simulink library "UAVdesign_net"  (Simulink 7.7)
settings: Solver=ode45  SolverMode=SingleTasking  StartTime=0.0  StopTime=10.0  RelTol=1e-3
undefined symbols (not defined in the file or in its folder): alpha_IERA_IELA_IELA, R_IERA_RA_RA
libraries: UAVdesign_net x75, simulink x13
(part 7 of 8)

== system UAVdesign_net/Vehicle Models/Helicopter Model/RA to IELA CG computation/RA to IELA 4 ==
  Geometry : Inport  OutDataTypeStr=Bus: GeometryParameters
  CG_RA_RA : Inport  Port=2
  Bus Selector : BusSelector  OutputSignals=R_IERA_RA_RA,alpha_IERA_IELA_IELA,m,I_IERA
  Dot Product : simulink/Math Operations/Dot Product  InputSameDT=on  OutDataType=sfix(16)  OutScaling=2^-10  DoSatur=off
  Identity matrix : Constant  Value=[1 0 0; 0 1 0; 0 0 1]
  Product : Product  RndMeth=Zero
  Product1 : Product  RndMeth=Zero
  Product2 : Product  Multiplication=Matrix(*)  RndMeth=Zero
  Product3 : Product  RndMeth=Zero
  RA to IELA1 : Subsystem
  Reshape : Reshape  OutputDimensionality=Column vector (2-D)
  Reshape1 : Reshape  OutputDimensionality=Row vector (2-D)
  Rotate to IELA : Product  Inputs=3  Multiplication=Matrix(*)  RndMeth=Zero
  Rotation Matrix from IELA to IERA : UAVdesign_net/Utilities/Axes/Euler Rotation Matrix from Earth to Body  SystemSampleTime=-1
  Sum : Sum  Inputs=-+|
  Sum1 : Sum  Inputs=+|+
  Sum2 : Sum  Inputs=|+-
  Transpose : Subsystem
      mask Display: disp('A^T', 'texmode', 'on')
  R_IELA_B_B : Outport
  alpha_IERA_IELA : Outport  Port=2
  T_IERA_IELA : Outport  Port=3
  T_IELA_IERA : Outport  Port=4
  mass_distance : Outport  Port=5
  m : Outport  Port=6
  In_CG : Outport  Port=7
  wires:
  Bus Selector/4 -> Rotate to IELA/2  "<I_IERA>"
  Rotate to IELA/1 -> Sum1/1
  Transpose/1(Out) -> Rotate to IELA/3, T_IELA_IERA/1
  Rotation Matrix from IELA to IERA/1 -> Rotate to IELA/1, T_IERA_IELA/1, Transpose/1(In)
  RA to IELA1/1(IELA) -> R_IELA_B_B/1, Reshape/1, Reshape1/1, Dot Product/2, Dot Product/1
  CG_RA_RA/1 -> Sum/1
  Sum1/1 -> In_CG/1
  Product/1 -> mass_distance/1
  Geometry/1 -> Bus Selector/1
  Sum2/1 -> Product1/2
  Product2/1 -> Sum2/2
  Product3/1 -> Sum2/1
  Identity matrix/1 -> Product3/1
  Dot Product/1 -> Product3/2
  Reshape1/1 -> Product2/2
  Reshape/1 -> Product2/1
  Product1/1 -> Sum1/2
  Sum/1 -> RA to IELA1/1(RA)
  Bus Selector/3 -> m/1, Product1/1, Product/2  "<m>"
  Bus Selector/2 -> Rotation Matrix from IELA to IERA/1, alpha_IERA_IELA/1  "<alpha_IERA_IELA_IELA>"
  Bus Selector/1 -> Sum/2, Product/1  "<R_IERA_RA_RA>"

== system UAVdesign_net/Vehicle Models/Helicopter Model/RA to IELA CG computation/RA to IELA 5 ==
  Geometry : Inport  OutDataTypeStr=Bus: GeometryParameters
  CG_RA_RA : Inport  Port=2
  Bus Selector : BusSelector  OutputSignals=R_IERA_RA_RA,alpha_IERA_IELA_IELA,m,I_IERA
  Dot Product : simulink/Math Operations/Dot Product  InputSameDT=on  OutDataType=sfix(16)  OutScaling=2^-10  DoSatur=off
  Identity matrix : Constant  Value=[1 0 0; 0 1 0; 0 0 1]
  Product : Product  RndMeth=Zero
  Product1 : Product  RndMeth=Zero
  Product2 : Product  Multiplication=Matrix(*)  RndMeth=Zero
  Product3 : Product  RndMeth=Zero
  RA to IELA1 : Subsystem
  Reshape : Reshape  OutputDimensionality=Column vector (2-D)
  Reshape1 : Reshape  OutputDimensionality=Row vector (2-D)
  Rotate to IELA : Product  Inputs=3  Multiplication=Matrix(*)  RndMeth=Zero
  Rotation Matrix from IELA to IERA : UAVdesign_net/Utilities/Axes/Euler Rotation Matrix from Earth to Body  SystemSampleTime=-1
  Sum : Sum  Inputs=-+|
  Sum1 : Sum  Inputs=+|+
  Sum2 : Sum  Inputs=|+-
  Transpose : Subsystem
      mask Display: disp('A^T', 'texmode', 'on')
  R_IELA_B_B : Outport
  alpha_IERA_IELA : Outport  Port=2
  T_IERA_IELA : Outport  Port=3
  T_IELA_IERA : Outport  Port=4
  mass_distance : Outport  Port=5
  m : Outport  Port=6
  In_CG : Outport  Port=7
  wires:
  Bus Selector/1 -> Product/1, Sum/2  "<R_IERA_RA_RA>"
  Bus Selector/2 -> alpha_IERA_IELA/1, Rotation Matrix from IELA to IERA/1  "<alpha_IERA_IELA_IELA>"
  Bus Selector/3 -> Product/2, Product1/1, m/1  "<m>"
  Sum/1 -> RA to IELA1/1(RA)
  Product1/1 -> Sum1/2
  Reshape/1 -> Product2/1
  Reshape1/1 -> Product2/2
  Dot Product/1 -> Product3/2
  Identity matrix/1 -> Product3/1
  Product3/1 -> Sum2/1
  Product2/1 -> Sum2/2
  Sum2/1 -> Product1/2
  Geometry/1 -> Bus Selector/1
  Product/1 -> mass_distance/1
  Sum1/1 -> In_CG/1
  CG_RA_RA/1 -> Sum/1
  RA to IELA1/1(IELA) -> Dot Product/1, Dot Product/2, Reshape1/1, Reshape/1, R_IELA_B_B/1
  Rotation Matrix from IELA to IERA/1 -> Transpose/1(In), T_IERA_IELA/1, Rotate to IELA/1
  Transpose/1(Out) -> T_IELA_IERA/1, Rotate to IELA/3
  Rotate to IELA/1 -> Sum1/1
  Bus Selector/4 -> Rotate to IELA/2  "<I_IERA>"

== system UAVdesign_net/Vehicle Models/Helicopter Model/RA to IELA CG computation/RA to IELA 6 ==
  Geometry : Inport  OutDataTypeStr=Bus: GeometryParameters
  CG_RA_RA : Inport  Port=2
  Bus Selector : BusSelector  OutputSignals=R_IERA_RA_RA,alpha_IERA_IELA_IELA,m,I_IERA
  Dot Product : simulink/Math Operations/Dot Product  InputSameDT=on  OutDataType=sfix(16)  OutScaling=2^-10  DoSatur=off
  Identity matrix : Constant  Value=[1 0 0; 0 1 0; 0 0 1]
  Product : Product  RndMeth=Zero
  Product1 : Product  RndMeth=Zero
  Product2 : Product  Multiplication=Matrix(*)  RndMeth=Zero
  Product3 : Product  RndMeth=Zero
  RA to IELA1 : Subsystem
  Reshape : Reshape  OutputDimensionality=Column vector (2-D)
  Reshape1 : Reshape  OutputDimensionality=Row vector (2-D)
  Rotate to IELA : Product  Inputs=3  Multiplication=Matrix(*)  RndMeth=Zero
  Rotation Matrix from IELA to IERA : UAVdesign_net/Utilities/Axes/Euler Rotation Matrix from Earth to Body  SystemSampleTime=-1
  Sum : Sum  Inputs=-+|
  Sum1 : Sum  Inputs=+|+
  Sum2 : Sum  Inputs=|+-
  Transpose : Subsystem
      mask Display: disp('A^T', 'texmode', 'on')
  R_IELA_B_B : Outport
  alpha_IERA_IELA : Outport  Port=2
  T_IERA_IELA : Outport  Port=3
  T_IELA_IERA : Outport  Port=4
  mass_distance : Outport  Port=5
  m : Outport  Port=6
  In_CG : Outport  Port=7
  wires:
  Bus Selector/4 -> Rotate to IELA/2  "<I_IERA>"
  Rotate to IELA/1 -> Sum1/1
  Transpose/1(Out) -> Rotate to IELA/3, T_IELA_IERA/1
  Rotation Matrix from IELA to IERA/1 -> Rotate to IELA/1, T_IERA_IELA/1, Transpose/1(In)
  RA to IELA1/1(IELA) -> R_IELA_B_B/1, Reshape/1, Reshape1/1, Dot Product/2, Dot Product/1
  CG_RA_RA/1 -> Sum/1
  Sum1/1 -> In_CG/1
  Product/1 -> mass_distance/1
  Geometry/1 -> Bus Selector/1
  Sum2/1 -> Product1/2
  Product2/1 -> Sum2/2
  Product3/1 -> Sum2/1
  Identity matrix/1 -> Product3/1
  Dot Product/1 -> Product3/2
  Reshape1/1 -> Product2/2
  Reshape/1 -> Product2/1
  Product1/1 -> Sum1/2
  Sum/1 -> RA to IELA1/1(RA)
  Bus Selector/3 -> m/1, Product1/1, Product/2  "<m>"
  Bus Selector/2 -> Rotation Matrix from IELA to IERA/1, alpha_IERA_IELA/1  "<alpha_IERA_IELA_IELA>"
  Bus Selector/1 -> Sum/2, Product/1  "<R_IERA_RA_RA>"

== system UAVdesign_net/Vehicle Models/Quad-Rotor Model (Momentum)/Fuselage/CG to IELA ==
  R_IELA-B|B : Inport
  V_B-E|B : Inport  Port=2
  omega_B_E|B : Inport  Port=3
  3x3 Cross Product : UAVdesign_net/Utilities/Math/3x3 Cross Product  SystemSampleTime=-1
  Sum : Sum  Inputs=++|
  V_IELA-E|IELA : Outport
  omega_IELA-E|IELA : Outport  Port=2
  wires:
  Sum/1 -> V_IELA-E|IELA/1
  V_B-E|B/1 -> Sum/1
  3x3 Cross Product/1 -> Sum/2
  R_IELA-B|B/1 -> 3x3 Cross Product/2
  omega_B_E|B/1 -> omega_IELA-E|IELA/1, 3x3 Cross Product/1

== system UAVdesign_net/Vehicle Models/Quad-Rotor Model (Momentum)/Fuselage/Fuselage Model (IERA) ==
  Parameters : Inport
  Environment : Inport  Port=2
  V_A : Inport  Port=3
  omega_A : Inport  Port=4
  V_W : Inport  Port=5
  omega_W : Inport  Port=6
  Fuselage Forces and Moments : Subsystem
      mask Display:
      | port_label('input', 1, 'Parameters', 'texmode', 'on')
      | port_label('input', 2, 'Environment', 'texmode', 'on')
      | port_label('input', 3, 'V_{A|WRA}', 'texmode', 'on')
      | port_label('input', 4, '\omega_{A|WRA}', 'texmode', 'on')
      | 
      | port_label('output', 1, 'FM_{A}', 'texmode', 'on')
  Fuselage Self-Influence : Subsystem
      mask Display:
      | port_label('input', 1, 'Parameters', 'texmode', 'on')
      | port_label('input', 2, 'Environment', 'texmode', 'on')
      | port_label('input', 3, 'V_{A|IERA}', 'texmode', 'on')
      | port_label('input', 4, '\omega_{A|IERA}', 'texmode', 'on')
      | port_label('input', 5, 'FM_{A|IERA}', 'texmode', 'on')
      | 
      | port_label('output', 1, 'd_{k|IERA}', 'texmode', 'on')
  Terminator : Terminator
  Terminator1 : Terminator
  Zero inertial : Constant  Value=[0 0 0 0 0 0]
  FM_I : Outport
  FM_A : Outport  Port=2
  d (k) : Outport  Port=3
  wires:
  Fuselage Self-Influence/1(d (k)) -> d (k)/1
  Fuselage Forces and Moments/1(FM_A) -> Fuselage Self-Influence/5(FM_A), FM_A/1
  Zero inertial/1 -> FM_I/1
  omega_W/1 -> Terminator1/1
  V_W/1 -> Terminator/1
  omega_A/1 -> Fuselage Forces and Moments/4(omega_A), Fuselage Self-Influence/4(omega_A)
  V_A/1 -> Fuselage Forces and Moments/3(V_A), Fuselage Self-Influence/3(V_A)
  Environment/1 -> Fuselage Forces and Moments/2(Environment), Fuselage Self-Influence/2(Environment)
  Parameters/1 -> Fuselage Forces and Moments/1(Parameters), Fuselage Self-Influence/1(Parameters)

== system UAVdesign_net/Vehicle Models/Quad-Rotor Model (Momentum)/Fuselage/IELA to CG ==
  R_IELA_B_B : Inport
  FM_IELA : Inport  Port=2
  3x3 Cross Product : UAVdesign_net/Utilities/Math/3x3 Cross Product  SystemSampleTime=-1
  Demux : Demux  Outputs=2
  Mux : Mux  Inputs=2
  Sum : Sum  Inputs=++|
  FM_B : Outport
  wires:
  3x3 Cross Product/1 -> Sum/1
  Sum/1 -> Mux/2
  Demux/2 -> Sum/2
  R_IELA_B_B/1 -> 3x3 Cross Product/1
  Demux/1 -> 3x3 Cross Product/2, Mux/1
  Mux/1 -> FM_B/1
  FM_IELA/1 -> Demux/1

== system UAVdesign_net/Vehicle Models/Quad-Rotor Model (Momentum)/Fuselage/IELA to IERA ==
  T_IERA_IELA : Inport
  V_A_IELA : Inport  Port=2
  omega_A_IELA : Inport  Port=3
  V_W_IELA : Inport  Port=4
  omega_W_IELA : Inport  Port=5
  1D : Reshape
  Demux : Demux
  Product : Product  Multiplication=Matrix(*)  RndMeth=Zero
  Vector Concatenate : Concatenate  NumInputs=4  Mode=Multidimensional array  ConcatenateDimension=2
  V_A_IERA : Outport
  omega_A_IERA : Outport  Port=2
  V_W_IERA : Outport  Port=3
  omega_W_IERA : Outport  Port=4
  wires:
  omega_W_IELA/1 -> Vector Concatenate/4
  V_W_IELA/1 -> Vector Concatenate/3
  Demux/4 -> omega_W_IERA/1
  Demux/3 -> V_W_IERA/1
  Demux/2 -> omega_A_IERA/1
  Demux/1 -> V_A_IERA/1
  1D/1 -> Demux/1
  Product/1 -> 1D/1
  Vector Concatenate/1 -> Product/2
  omega_A_IELA/1 -> Vector Concatenate/2
  V_A_IELA/1 -> Vector Concatenate/1
  T_IERA_IELA/1 -> Product/1

== system UAVdesign_net/Vehicle Models/Quad-Rotor Model (Momentum)/Fuselage/IERA to IELA ==
  T_IELA_IERA : Inport
  FM_I_IERA : Inport  Port=2
  FM_A_IERA : Inport  Port=3
  d_IERA : Inport  Port=4
  1D : Reshape
  Demux : Demux  Outputs=[6 6 3]
  Demux1 : Demux  Outputs=2
  Demux2 : Demux  Outputs=2
  Product : Product  Multiplication=Matrix(*)  RndMeth=Zero
  Signal Specification{,1..4} (5 alike) : SignalSpecification  Dimensions=3
  Vector Concatenate : Concatenate  NumInputs=5  Mode=Multidimensional array  ConcatenateDimension=2
  FM_I_IELA : Outport
  FM_A_IELA : Outport  Port=2
  d_IELA : Outport  Port=3
  wires:
  Signal Specification4/1 -> Vector Concatenate/5
  Signal Specification3/1 -> Vector Concatenate/4
  Signal Specification2/1 -> Vector Concatenate/3
  Signal Specification1/1 -> Vector Concatenate/2
  Signal Specification/1 -> Vector Concatenate/1
  FM_A_IERA/1 -> Demux2/1
  Demux2/2 -> Signal Specification3/1
  Demux2/1 -> Signal Specification2/1
  Demux1/1 -> Signal Specification/1
  Demux1/2 -> Signal Specification1/1
  FM_I_IERA/1 -> Demux1/1
  d_IERA/1 -> Signal Specification4/1
  Demux/3 -> d_IELA/1
  Demux/2 -> FM_A_IELA/1
  Demux/1 -> FM_I_IELA/1
  1D/1 -> Demux/1
  Product/1 -> 1D/1
  Vector Concatenate/1 -> Product/2
  T_IELA_IERA/1 -> Product/1

== system UAVdesign_net/Vehicle Models/Quad-Rotor Model (Momentum)/Fuselage/Transpose ==
  In : Inport
  Permute Dimensions : PermuteDimensions
  Out : Outport
  wires:
  In/1 -> Permute Dimensions/1
  Permute Dimensions/1 -> Out/1

== system UAVdesign_net/Vehicle Models/Quad-Rotor Model (Momentum)/RA to IELA CG computation/Body Coordinates Computation ==
  Geometry : Inport
  R_CG_RA_RA : Inport  Port=2
  Assignment : Assignment  NumberOfDimensions=2  IndexMode=Zero-based  OutputInitialize=Specify size for each dimension in table  IndexOptions=Assign all,Starting index (port)  Indices=1,1  OutputSizes=3,3*6
  Assignment1 : Assignment  IndexMode=Zero-based  OutputInitialize=Specify size for each dimension in table  IndexOptions=Starting index (port)  Indices=1  OutputSizes=3*6
  Bus Selector : BusSelector  OutputSignals=COMMON.R_IERA_RA_RA,COMMON.alpha_IERA_IELA_IELA,COMMON.m,COMMON.I_IERA
  For Iterator : ForIterator  ResetStates=reset  IterationLimit=6  IndexMode=Zero-based
  Gain{,1..4} (5 alike) : Gain  Gain=3  OutDataTypeStr=uint32
  RA to IELA : Subsystem
  Rotation Matrix from IELA to IERA : UAVdesign_net/Utilities/Axes/Euler Rotation Matrix from Earth to Body  SystemSampleTime=-1
  Selector : Selector  IndexMode=Zero-based  InputPortWidth=3*6  IndexOptions=Starting index (port)  Indices=[1 3]  OutputSizes=3
  Selector1 : Selector  IndexMode=Zero-based  InputPortWidth=3*6  IndexOptions=Starting index (port)  Indices=[1 3]  OutputSizes=3
  Selector2 : Selector  IndexMode=Zero-based  InputPortWidth=6  IndexOptions=Starting index (port)  Indices=[1 3]  OutputSizes=1
  Selector3 : Selector  NumberOfDimensions=2  IndexMode=Zero-based  InputPortWidth=6  IndexOptions=Select all,Starting index (port)  Indices=[1 3],1  OutputSizes=1,3
  Sum : Sum  Inputs=|++
  Unit Delay : UnitDelay  SampleTime=-1
  R_IERA_B_B : Outport
  T_IERA_IELA : Outport  Port=2
  Inb : Outport  Port=3
  wires:
  Sum/1 -> Unit Delay/1, Inb/1
  Unit Delay/1 -> Sum/1
  RA to IELA/2(In_CG) -> Sum/2
  Gain/1 -> Selector/2
  Gain1/1 -> Selector1/2
  For Iterator/1 -> Gain/1, Gain1/1, Selector2/2, Gain2/1, Gain3/1, Gain4/1
  Bus Selector/3 -> Selector2/1  "<m>"
  Geometry/1 -> Bus Selector/1
  Bus Selector/1 -> Selector/1  "<R_IERA_RA_RA>"
  Bus Selector/2 -> Selector1/1  "<alpha_IERA_IELA_IELA>"
  Rotation Matrix from IELA to IERA/1 -> RA to IELA/5(T_IERA_IELA), Assignment/1
  Bus Selector/4 -> Selector3/1  "<I_IERA>"
  Gain2/1 -> Selector3/2
  Selector1/1 -> Rotation Matrix from IELA to IERA/1
  Selector3/1 -> RA to IELA/4(I_IERA)
  Selector2/1 -> RA to IELA/3(m)
  Selector/1 -> RA to IELA/2(R_IERA_RA_RA)
  R_CG_RA_RA/1 -> RA to IELA/1(R_CG_RA_RA)
  Assignment/1 -> T_IERA_IELA/1
  Gain3/1 -> Assignment/2
  Gain4/1 -> Assignment1/2
  Assignment1/1 -> R_IERA_B_B/1
  RA to IELA/1(R_IELA_B_B) -> Assignment1/1

== system UAVdesign_net/Vehicle Models/Quad-Rotor Model (Momentum)/RA to IELA CG computation/GC Computation ==
  Geometry : Inport
  Bus Selector : BusSelector  OutputSignals=COMMON.R_IERA_RA_RA,COMMON.m
  For Iterator : ForIterator  ResetStates=reset  IterationLimit=6  IndexMode=Zero-based
  Gain : Gain  Gain=3  OutDataTypeStr=uint32
  Product : Product  RndMeth=Zero
  Selector : Selector  IndexMode=Zero-based  InputPortWidth=3*6  IndexOptions=Starting index (port)  Indices=[1 3]  OutputSizes=3
  Selector2 : Selector  IndexMode=Zero-based  InputPortWidth=6  IndexOptions=Starting index (port)  Indices=[1 3]  OutputSizes=1
  Sum : Sum  Inputs=|++
  Sum2 : Sum  Inputs=|++
  Unit Delay : UnitDelay  SampleTime=-1
  Unit Delay2 : UnitDelay  X0=[0 0 0]  SampleTime=-1
  R_CG_RA_RA_m : Outport
  mass : Outport  Port=2
  wires:
  Unit Delay/1 -> Sum/1
  Sum/1 -> mass/1, Unit Delay/1
  Unit Delay2/1 -> Sum2/1
  Sum2/1 -> Unit Delay2/1, R_CG_RA_RA_m/1
  Product/1 -> Sum2/2
  Selector2/1 -> Sum/2, Product/2
  Selector/1 -> Product/1
  Gain/1 -> Selector/2
  For Iterator/1 -> Gain/1, Selector2/2
  Bus Selector/2 -> Selector2/1  "<m>"
  Geometry/1 -> Bus Selector/1
  Bus Selector/1 -> Selector/1  "<R_IERA_RA_RA>"

== system UAVdesign_net/Subsystem Models/Fin/Fin Model (IERA)/Fin/Fin Forces and Moments ==
  Parameters : Inport  OutDataTypeStr=Bus: FinParameters
  Environment : Inport  Port=2  OutDataTypeStr=Bus: Environment
  V_A : Inport  Port=3
  omega_A : Inport  Port=4
  Fin Forces and Moments (WRA axes) : Stateflow chart  TreatAsAtomicUnit=on
  FM_A : Outport
  wires:
  Parameters/1 -> Fin Forces and Moments (WRA axes)/1(Parameters)
  Environment/1 -> Fin Forces and Moments (WRA axes)/2(Environment)
  V_A/1 -> Fin Forces and Moments (WRA axes)/3(va)
  omega_A/1 -> Fin Forces and Moments (WRA axes)/4(oma)
  Fin Forces and Moments (WRA axes)/1(FM_A) -> FM_A/1

== system UAVdesign_net/Subsystem Models/Fin/Fin Model (IERA)/Fin/IERA to MAC ==
  R_xW-IERA|IERA : Inport
  V_A|IERA : Inport  Port=2
  omega_A|IERA : Inport  Port=3
  3x3 Cross Product : UAVdesign_net/Utilities/Math/3x3 Cross Product  SystemSampleTime=-1
  Sum : Sum  Inputs=++|
  V_A|MAC : Outport
  omega_A|MAC : Outport  Port=2
  wires:
  Sum/1 -> V_A|MAC/1
  V_A|IERA/1 -> Sum/1
  3x3 Cross Product/1 -> Sum/2
  R_xW-IERA|IERA/1 -> 3x3 Cross Product/2
  omega_A|IERA/1 -> omega_A|MAC/1, 3x3 Cross Product/1

== system UAVdesign_net/Subsystem Models/Fin/Fin Model (IERA)/Fin/MAC to IERA ==
  R_MAC_IERA_IERA : Inport
  FM_MAC : Inport  Port=2
  3x3 Cross Product : UAVdesign_net/Utilities/Math/3x3 Cross Product  SystemSampleTime=-1
  Demux : Demux  Outputs=2
  Mux : Mux  Inputs=2
  Sum : Sum  Inputs=++|
  FM_IERA : Outport
  wires:
  FM_MAC/1 -> Demux/1
  Mux/1 -> FM_IERA/1
  Demux/1 -> Mux/1, 3x3 Cross Product/2
  R_MAC_IERA_IERA/1 -> 3x3 Cross Product/1
  Demux/2 -> Sum/2
  Sum/1 -> Mux/2
  3x3 Cross Product/1 -> Sum/1

== system UAVdesign_net/Subsystem Models/Fin/Fin Model (IERA)/Fin/MAC to WRA (Half Wing) ==
  T_WRA_MAC : Inport
  V_A_MAC : Inport  Port=2
  omega_A_MAC : Inport  Port=3
  1D : Reshape
  Demux : Demux  Outputs=2
  Product : Product  Multiplication=Matrix(*)  RndMeth=Zero
  Vector Concatenate : Concatenate  Mode=Multidimensional array  ConcatenateDimension=2
  V_A_WRA : Outport
  omega_A_WRA : Outport  Port=2
  wires:
  Demux/2 -> omega_A_WRA/1
  Demux/1 -> V_A_WRA/1
  1D/1 -> Demux/1
  Product/1 -> 1D/1
  Vector Concatenate/1 -> Product/2
  omega_A_MAC/1 -> Vector Concatenate/2
  V_A_MAC/1 -> Vector Concatenate/1
  T_WRA_MAC/1 -> Product/1

== system UAVdesign_net/Subsystem Models/Fin/Fin Model (IERA)/Fin/WRA to MAC ==
  T_IERA_WM : Inport
  FM_A_WM : Inport  Port=2
  1D : Reshape
  Demux1 : Demux  Outputs=2
  Product : Product  Multiplication=Matrix(*)  RndMeth=Zero
  Vector Concatenate : Concatenate  Mode=Multidimensional array  ConcatenateDimension=2
  FM_A_IERA : Outport
  wires:
  T_IERA_WM/1 -> Product/1
  Vector Concatenate/1 -> Product/2
  Product/1 -> 1D/1
  1D/1 -> FM_A_IERA/1
  Demux1/1 -> Vector Concatenate/1
  Demux1/2 -> Vector Concatenate/2
  FM_A_WM/1 -> Demux1/1

== system UAVdesign_net/Subsystem Models/Wing/Wing Model (IERA)/Left Wing/Half Wing Forces and Moments ==
  Parameters : Inport  OutDataTypeStr=Bus: FinParameters
  Environment : Inport  Port=2  OutDataTypeStr=Bus: Environment
  V_A : Inport  Port=3
  omega_A : Inport  Port=4
  Wing Forces and Moments (WRA axes) : Stateflow chart  TreatAsAtomicUnit=on
  FM_A : Outport
  wires:
  Parameters/1 -> Wing Forces and Moments (WRA axes)/1(Parameters)
  Environment/1 -> Wing Forces and Moments (WRA axes)/2(Environment)
  V_A/1 -> Wing Forces and Moments (WRA axes)/3(va)
  omega_A/1 -> Wing Forces and Moments (WRA axes)/4(oma)
  Wing Forces and Moments (WRA axes)/1(FM_A) -> FM_A/1

== system UAVdesign_net/Subsystem Models/Wing/Wing Model (IERA)/Left Wing/IERA to MAC ==
  R_xW-IERA|IERA : Inport
  V_A|IERA : Inport  Port=2
  omega_A|IERA : Inport  Port=3
  3x3 Cross Product : UAVdesign_net/Utilities/Math/3x3 Cross Product  SystemSampleTime=-1
  Sum : Sum  Inputs=++|
  V_A|MAC : Outport
  omega_A|MAC : Outport  Port=2
  wires:
  Sum/1 -> V_A|MAC/1
  V_A|IERA/1 -> Sum/1
  3x3 Cross Product/1 -> Sum/2
  R_xW-IERA|IERA/1 -> 3x3 Cross Product/2
  omega_A|IERA/1 -> omega_A|MAC/1, 3x3 Cross Product/1

== system UAVdesign_net/Subsystem Models/Wing/Wing Model (IERA)/Left Wing/MAC to IERA ==
  R_MAC_IERA_IERA : Inport
  FM_MAC : Inport  Port=2
  3x3 Cross Product : UAVdesign_net/Utilities/Math/3x3 Cross Product  SystemSampleTime=-1
  Demux : Demux  Outputs=2
  Mux : Mux  Inputs=2
  Sum : Sum  Inputs=++|
  FM_IERA : Outport
  wires:
  FM_MAC/1 -> Demux/1
  Mux/1 -> FM_IERA/1
  Demux/1 -> Mux/1, 3x3 Cross Product/2
  R_MAC_IERA_IERA/1 -> 3x3 Cross Product/1
  Demux/2 -> Sum/2
  Sum/1 -> Mux/2
  3x3 Cross Product/1 -> Sum/1

== system UAVdesign_net/Subsystem Models/Wing/Wing Model (IERA)/Left Wing/MAC to WRA (Half Wing) ==
  T_WRA_MAC : Inport
  V_A_MAC : Inport  Port=2
  omega_A_MAC : Inport  Port=3
  1D : Reshape
  Demux : Demux  Outputs=2
  Product : Product  Multiplication=Matrix(*)  RndMeth=Zero
  Vector Concatenate : Concatenate  Mode=Multidimensional array  ConcatenateDimension=2
  V_A_WRA : Outport
  omega_A_WRA : Outport  Port=2
  wires:
  Demux/2 -> omega_A_WRA/1
  Demux/1 -> V_A_WRA/1
  1D/1 -> Demux/1
  Product/1 -> 1D/1
  Vector Concatenate/1 -> Product/2
  omega_A_MAC/1 -> Vector Concatenate/2
  V_A_MAC/1 -> Vector Concatenate/1
  T_WRA_MAC/1 -> Product/1

== system UAVdesign_net/Subsystem Models/Wing/Wing Model (IERA)/Left Wing/WRA to MAC ==
  T_IERA_WM : Inport
  FM_A_WM : Inport  Port=2
  1D : Reshape
  Demux1 : Demux  Outputs=2
  Product : Product  Multiplication=Matrix(*)  RndMeth=Zero
  Vector Concatenate : Concatenate  Mode=Multidimensional array  ConcatenateDimension=2
  FM_A_IERA : Outport
  wires:
  T_IERA_WM/1 -> Product/1
  Vector Concatenate/1 -> Product/2
  Product/1 -> 1D/1
  1D/1 -> FM_A_IERA/1
  Demux1/1 -> Vector Concatenate/1
  Demux1/2 -> Vector Concatenate/2
  FM_A_WM/1 -> Demux1/1

== system UAVdesign_net/Subsystem Models/Wing/Wing Model (IERA)/Right Wing/Half Wing Forces and Moments ==
  Parameters : Inport  OutDataTypeStr=Bus: FinParameters
  Environment : Inport  Port=2  OutDataTypeStr=Bus: Environment
  V_A : Inport  Port=3
  omega_A : Inport  Port=4
  Wing Forces and Moments (WRA axes) : Stateflow chart  TreatAsAtomicUnit=on
  FM_A : Outport
  wires:
  Wing Forces and Moments (WRA axes)/1(FM_A) -> FM_A/1
  omega_A/1 -> Wing Forces and Moments (WRA axes)/4(oma)
  V_A/1 -> Wing Forces and Moments (WRA axes)/3(va)
  Environment/1 -> Wing Forces and Moments (WRA axes)/2(Environment)
  Parameters/1 -> Wing Forces and Moments (WRA axes)/1(Parameters)

== system UAVdesign_net/Subsystem Models/Wing/Wing Model (IERA)/Right Wing/IERA to MAC ==
  R_xW-IERA|IERA : Inport
  V_A|IERA : Inport  Port=2
  omega_A|IERA : Inport  Port=3
  3x3 Cross Product : UAVdesign_net/Utilities/Math/3x3 Cross Product  SystemSampleTime=-1
  Sum : Sum  Inputs=++|
  V_A|MAC : Outport
  omega_A|MAC : Outport  Port=2
  wires:
  omega_A|IERA/1 -> 3x3 Cross Product/1, omega_A|MAC/1
  R_xW-IERA|IERA/1 -> 3x3 Cross Product/2
  3x3 Cross Product/1 -> Sum/2
  V_A|IERA/1 -> Sum/1
  Sum/1 -> V_A|MAC/1

== system UAVdesign_net/Subsystem Models/Wing/Wing Model (IERA)/Right Wing/MAC to IERA ==
  R_MAC_IERA_IERA : Inport
  FM_MAC : Inport  Port=2
  3x3 Cross Product : UAVdesign_net/Utilities/Math/3x3 Cross Product  SystemSampleTime=-1
  Demux : Demux  Outputs=2
  Mux : Mux  Inputs=2
  Sum : Sum  Inputs=++|
  FM_IERA : Outport
  wires:
  3x3 Cross Product/1 -> Sum/1
  Sum/1 -> Mux/2
  Demux/2 -> Sum/2
  R_MAC_IERA_IERA/1 -> 3x3 Cross Product/1
  Demux/1 -> 3x3 Cross Product/2, Mux/1
  Mux/1 -> FM_IERA/1
  FM_MAC/1 -> Demux/1

== system UAVdesign_net/Subsystem Models/Wing/Wing Model (IERA)/Right Wing/MAC to WRA (Half Wing) ==
  T_WRA_MAC : Inport
  V_A_MAC : Inport  Port=2
  omega_A_MAC : Inport  Port=3
  1D : Reshape
  Demux : Demux  Outputs=2
  Product : Product  Multiplication=Matrix(*)  RndMeth=Zero
  Vector Concatenate : Concatenate  Mode=Multidimensional array  ConcatenateDimension=2
  V_A_WRA : Outport
  omega_A_WRA : Outport  Port=2
  wires:
  T_WRA_MAC/1 -> Product/1
  V_A_MAC/1 -> Vector Concatenate/1
  omega_A_MAC/1 -> Vector Concatenate/2
  Vector Concatenate/1 -> Product/2
  Product/1 -> 1D/1
  1D/1 -> Demux/1
  Demux/1 -> V_A_WRA/1
  Demux/2 -> omega_A_WRA/1

== system UAVdesign_net/Subsystem Models/Wing/Wing Model (IERA)/Right Wing/WRA to MAC ==
  T_IERA_WM : Inport
  FM_A_WM : Inport  Port=2
  1D : Reshape
  Demux1 : Demux  Outputs=2
  Product : Product  Multiplication=Matrix(*)  RndMeth=Zero
  Vector Concatenate : Concatenate  Mode=Multidimensional array  ConcatenateDimension=2
  FM_A_IERA : Outport
  wires:
  FM_A_WM/1 -> Demux1/1
  Demux1/2 -> Vector Concatenate/2
  Demux1/1 -> Vector Concatenate/1
  1D/1 -> FM_A_IERA/1
  Product/1 -> 1D/1
  Vector Concatenate/1 -> Product/2
  T_IERA_WM/1 -> Product/1

== system UAVdesign_net/Vehicle Models/Helicopter Model/RA to IELA CG computation/RA to IELA/RA to IELA1 ==
  RA : Inport
  Constant1 : Constant  Value=[-1 1 -1]
  Product : Product  RndMeth=Zero
  IELA : Outport
  wires:
  Constant1/1 -> Product/1
  Product/1 -> IELA/1
  RA/1 -> Product/2

== system UAVdesign_net/Vehicle Models/Helicopter Model/RA to IELA CG computation/RA to IELA/Transpose ==
  In : Inport
  Permute Dimensions : PermuteDimensions
  Out : Outport
  wires:
  Permute Dimensions/1 -> Out/1
  In/1 -> Permute Dimensions/1

== system UAVdesign_net/Vehicle Models/Helicopter Model/RA to IELA CG computation/RA to IELA 2/RA to IELA1 ==
  RA : Inport
  Constant1 : Constant  Value=[-1 1 -1]
  Product : Product  RndMeth=Zero
  IELA : Outport
  wires:
  RA/1 -> Product/2
  Product/1 -> IELA/1
  Constant1/1 -> Product/1

== system UAVdesign_net/Vehicle Models/Helicopter Model/RA to IELA CG computation/RA to IELA 2/Transpose ==
  In : Inport
  Permute Dimensions : PermuteDimensions
  Out : Outport
  wires:
  In/1 -> Permute Dimensions/1
  Permute Dimensions/1 -> Out/1

== system UAVdesign_net/Vehicle Models/Helicopter Model/RA to IELA CG computation/RA to IELA 3/RA to IELA1 ==
  RA : Inport
  Constant1 : Constant  Value=[-1 1 -1]
  Product : Product  RndMeth=Zero
  IELA : Outport
  wires:
  Constant1/1 -> Product/1
  Product/1 -> IELA/1
  RA/1 -> Product/2

== system UAVdesign_net/Vehicle Models/Helicopter Model/RA to IELA CG computation/RA to IELA 3/Transpose ==
  In : Inport
  Permute Dimensions : PermuteDimensions
  Out : Outport
  wires:
  Permute Dimensions/1 -> Out/1
  In/1 -> Permute Dimensions/1

== system UAVdesign_net/Vehicle Models/Helicopter Model/RA to IELA CG computation/RA to IELA 4/RA to IELA1 ==
  RA : Inport
  Constant1 : Constant  Value=[-1 1 -1]
  Product : Product  RndMeth=Zero
  IELA : Outport
  wires:
  RA/1 -> Product/2
  Product/1 -> IELA/1
  Constant1/1 -> Product/1

== system UAVdesign_net/Vehicle Models/Helicopter Model/RA to IELA CG computation/RA to IELA 4/Transpose ==
  In : Inport
  Permute Dimensions : PermuteDimensions
  Out : Outport
  wires:
  In/1 -> Permute Dimensions/1
  Permute Dimensions/1 -> Out/1

== system UAVdesign_net/Vehicle Models/Helicopter Model/RA to IELA CG computation/RA to IELA 5/RA to IELA1 ==
  RA : Inport
  Constant1 : Constant  Value=[-1 1 -1]
  Product : Product  RndMeth=Zero
  IELA : Outport
  wires:
  Constant1/1 -> Product/1
  Product/1 -> IELA/1
  RA/1 -> Product/2

== system UAVdesign_net/Vehicle Models/Helicopter Model/RA to IELA CG computation/RA to IELA 5/Transpose ==
  In : Inport
  Permute Dimensions : PermuteDimensions
  Out : Outport
  wires:
  Permute Dimensions/1 -> Out/1
  In/1 -> Permute Dimensions/1

== system UAVdesign_net/Vehicle Models/Helicopter Model/RA to IELA CG computation/RA to IELA 6/RA to IELA1 ==
  RA : Inport
  Constant1 : Constant  Value=[-1 1 -1]
  Product : Product  RndMeth=Zero
  IELA : Outport
  wires:
  RA/1 -> Product/2
  Product/1 -> IELA/1
  Constant1/1 -> Product/1

== system UAVdesign_net/Vehicle Models/Helicopter Model/RA to IELA CG computation/RA to IELA 6/Transpose ==
  In : Inport
  Permute Dimensions : PermuteDimensions
  Out : Outport
  wires:
  In/1 -> Permute Dimensions/1
  Permute Dimensions/1 -> Out/1

== system UAVdesign_net/Vehicle Models/Quad-Rotor Model (Momentum)/Fuselage/Fuselage Model (IERA)/Fuselage Forces and Moments ==
  Parameters : Inport
  Environment : Inport  Port=2
  V_A : Inport  Port=3
  omega_A : Inport  Port=4
  Fuselage Forces and Moments : Stateflow chart  TreatAsAtomicUnit=on
  FM_A : Outport
  wires:
  Parameters/1 -> Fuselage Forces and Moments/1(Parameters)
  Environment/1 -> Fuselage Forces and Moments/2(Environment)
  V_A/1 -> Fuselage Forces and Moments/3(va)
  omega_A/1 -> Fuselage Forces and Moments/4(oma)
  Fuselage Forces and Moments/1(FM_A) -> FM_A/1

== system UAVdesign_net/Vehicle Models/Quad-Rotor Model (Momentum)/Fuselage/Fuselage Model (IERA)/Fuselage Self-Influence ==
  Parameters : Inport
  Environment : Inport  Port=2
  V_A : Inport  Port=3
  omega_A : Inport  Port=4
  FM_A : Inport  Port=5
  Fuselage Wash Self-Influence : Stateflow chart  TreatAsAtomicUnit=on
  d (k) : Outport
  wires:
  Parameters/1 -> Fuselage Wash Self-Influence/1(Parameters)
  Fuselage Wash Self-Influence/1(d) -> d (k)/1
  Environment/1 -> Fuselage Wash Self-Influence/2(Environment)
  V_A/1 -> Fuselage Wash Self-Influence/3(va)
  omega_A/1 -> Fuselage Wash Self-Influence/4(oma)
  FM_A/1 -> Fuselage Wash Self-Influence/5(FM_A)

== system UAVdesign_net/Vehicle Models/Quad-Rotor Model (Momentum)/RA to IELA CG computation/Body Coordinates Computation/RA to IELA ==
  R_CG_RA_RA : Inport
  R_IERA_RA_RA : Inport  Port=2
  m : Inport  Port=3
  I_IERA : Inport  Port=4
  T_IERA_IELA : Inport  Port=5
  Dot Product : simulink/Math Operations/Dot Product  InputSameDT=on  OutDataType=sfix(16)  OutScaling=2^-10  DoSatur=off
  Identity matrix : Constant  Value=[1 0 0; 0 1 0; 0 0 1]
  Product1 : Product  RndMeth=Zero
  Product2 : Product  Multiplication=Matrix(*)  RndMeth=Zero
  Product3 : Product  RndMeth=Zero
  RA to IELA1 : Subsystem
  Reshape : Reshape  OutputDimensionality=Column vector (2-D)
  Reshape1 : Reshape  OutputDimensionality=Row vector (2-D)
  Rotate to IELA : Product  Inputs=3  Multiplication=Matrix(*)  RndMeth=Zero
  Sum : Sum  Inputs=-+|
  Sum1 : Sum  Inputs=+|+
  Sum2 : Sum  Inputs=|+-
  Transpose : UAVdesign_net/Utilities/Math/Transpose  SystemSampleTime=-1
  R_IELA_B_B : Outport
  In_CG : Outport  Port=2
  wires:
  Sum/1 -> RA to IELA1/1(RA)
  Product1/1 -> Sum1/2
  Reshape/1 -> Product2/1
  Reshape1/1 -> Product2/2
  Dot Product/1 -> Product3/2
  Identity matrix/1 -> Product3/1
  Product3/1 -> Sum2/1
  Product2/1 -> Sum2/2
  Sum2/1 -> Product1/2
  Sum1/1 -> In_CG/1
  R_CG_RA_RA/1 -> Sum/1
  RA to IELA1/1(IELA) -> Dot Product/1, Dot Product/2, Reshape1/1, Reshape/1, R_IELA_B_B/1
  Rotate to IELA/1 -> Sum1/1
  T_IERA_IELA/1 -> Rotate to IELA/1, Transpose/1
  Transpose/1 -> Rotate to IELA/3
  R_IERA_RA_RA/1 -> Sum/2
  I_IERA/1 -> Rotate to IELA/2
  m/1 -> Product1/1

== system UAVdesign_net/Vehicle Models/Quad-Rotor Model (Momentum)/RA to IELA CG computation/Body Coordinates Computation/RA to IELA/RA to IELA1 ==
  RA : Inport
  Constant1 : Constant  Value=[-1 1 -1]
  Product : Product  RndMeth=Zero
  IELA : Outport
  wires:
  Constant1/1 -> Product/1
  Product/1 -> IELA/1
  RA/1 -> Product/2

== matlab function Vehicle Models/Helicopter Model/Wash Coupling/Wash Coupling ==
  data: d input double; vw_omw output double; R input double; MR_radius input double size=1
function vw_omw  = wash_coupling(d, R, MR_radius)
% This block supports the Embedded MATLAB subset.
% See the help menu for details. 

MR =   1:3;
TR =   4:6;
FUSE = 7:9;
HW   = 10:12;
VF   = 13:15;

MRv =   1:3;
TRv =   7:9;
FUSEv = 13:15;
HWv   = 19:21;
VFv   = 25:27;
vw_omw = zeros(30,1);

% Self-influence
vw_omw(MRv) = d(MR);
vw_omw(TRv) = d(TR);
vw_omw(FUSEv) = zeros(3,1);  % the fuselage model already has the self-influence included
vw_omw(HWv) = d(HW);
vw_omw(VFv) = d(VF);

% Main rotor on fuselage
dist = sqrt((R(MR) - R(FUSE))' * (R(MR) - R(FUSE)));
zor = dist / MR_radius;
coef1 = 1 + zor / sqrt(1 + zor^2);
vw_omw(FUSEv(3)) = vw_omw(FUSEv(3)) + coef1 * d(MR(3));

% Main rotor on horizontal stabilizer - assumes
% the horizontal stabilizer is always in the wake.
dist = sqrt((R(MR) - R(HW))' * (R(MR) - R(HW)));
zor = dist / MR_radius;
coef1 = 1 + zor / sqrt(1 + zor^2);
vw_omw(HWv(3)) = vw_omw(HWv(3)) + coef1 * d(MR(3));

% Fuselage on main rotor
vw_omw(MRv(3)) = vw_omw(MRv(3)) + d(FUSE(3));

% Vertical fin on tail rotor
vw_omw(TRv(2)) = vw_omw(TRv(2)) + d(VF(2));

% Tail rotor on vertical fin
vw_omw(VFv(2)) = vw_omw(VFv(2)) + d(TR(2));

% Fuselage on horizontal stabilizer
vw_omw(HWv(1)) = vw_omw(HWv(1)) + d(FUSE(1));

% no rotation wakes generated

== matlab function Utilities/Axes/Attitude Estimation/Embedded MATLAB Function ==
  data: Ri input double; q_opt output double; Bi input double; a input double
function q_opt = ESOQ2(Ri, Bi, a)
% Each vector input has to contain two vectors in a 3x2 format
% sum(a) must be equal to 1

n = size(Ri, 2);

for i=1:n,
    normRi2 = Ri(:,i)'*Ri(:,i);
    if normRi2
        Ri(:,i) = Ri(:,i) / sqrt(normRi2);
    end
    normBi2 = Bi(:,i)'*Bi(:,i);
    if normBi2
        Bi(:,i) = Bi(:,i) / sqrt(normBi2);
    end
end

B = zeros(3,3);
for i=1:n,
    B = B + a(i) * (Bi(:,i) * Ri(:,i)');
end

% rotation to avoid singularity
if B(1,1)+B(2,2)+B(3,3) < 0
    rot_axis = 0;
elseif  B(1,1)-B(2,2)-B(3,3) < 0
    rot_axis = 1;
    B = [B(:,1) -B(:,2) -B(:,3)];
elseif -B(1,1)+B(2,2)-B(3,3) < 0
    rot_axis = 2;
    B = [-B(:,1) B(:,2) -B(:,3)];
else
    rot_axis = 3;
    B = [-B(:,1) -B(:,2) B(:,3)];
end

z = [B(2,3)-B(3,2); B(3,1)-B(1,3); B(1,2)-B(2,1)];
S = B + B';
BB = cross(Bi(:,1), Bi(:,2));
RR = cross(Ri(:,1), Ri(:,2));
lambda_max = sqrt(a(1)^2 + a(2)^2 + 2*a(1)*a(2)*(Bi(:,1)'*Bi(:,2)*Ri(:,1)'*Ri(:,2)+sqrt(BB'*BB*RR'*RR)));
M = (trace(B)-lambda_max)*(S-(trace(B)+lambda_max)*eye(3,3)) - z*z';
E = zeros(3,3);
E(:,1) = cross(M(:,2), M(:,3));
E(:,2) = cross(M(:,3), M(:,1));
E(:,3) = cross(M(:,1), M(:,2));
ek = E(:,1);
if abs(E(2,2)) > abs(E(1,1)),
    ek = E(:,2);
    if abs(E(3,3)) > abs(E(2,2)),
        ek = E(:,3);
    end
elseif abs(E(3,3)) > abs(E(1,1)),
    ek = E(:,3);
end
q_opt = [z'*ek; (lambda_max-trace(B))*ek];

% reverse the rotation used to avoid the singularity
switch rot_axis
    case 1
        q_opt = [-q_opt(2)  q_opt(1) -q_opt(4)  q_opt(3)]';
    case 2
        q_opt = [-q_opt(3)  q_opt(4)  q_opt(1) -q_opt(2)]';
    case 3
        q_opt = [-q_opt(4) -q_opt(3)  q_opt(2)  q_opt(1)]';
end

if q_opt'*q_opt == 0,
    q_opt = [1 0 0 0]';
end
q_opt = q_opt/sqrt(q_opt'*q_opt);

== matlab function Utilities/Continuous/Remote Execution Code ==
  data: SignalID input double; ufin output double; u0 input double; xdes input double; xfin output double
  events: exec output FUNCTION_CALL_EVENT
function [ufin, xfin] = remote_exec(SignalID, u0, xdes)

% Modify this block according to your algorithm
%
% Example of using the remote signals to execute a Simulink subsystem
% multiple times under software control during every simulation step
% It implements a Newton-Raphson algorithm that requires the following
% operations at every simulation step:
%  1. Provide the inputs to the external subsystem (u)
%  2. Execute the external subsystem
%  3. Read the outputs of the external subsystem (x)
%  4. Calculate the Jacobian and the new inputs that have to be provided
%     to the external subsystem
%  5. Decide if it's time to stop. If not, go to step 2
% The outputs of the Embedded Matlab block are the final solution of the
% Newton-Raphson algorithm

% Consider a system with 4 inputs and 4 outputs
Nin  = 4;
Nout = 4;

% Number of iterations
Niter = 5;

% Numeric perturbation. Values have to be scaled correctly
du      = [1; 1; 1; 1];
jac     = zeros(Nout, Nin);
u       = zeros(Nin, 1);
x       = zeros(Nout,1);
xfin    = zeros(Nout,1);

% Newton-Raphson iterations
for i=1:Niter
    
    % find Jacobian
    index_in  = 1;
    while index_in <= Nin
        u = u0;
        u(index_in) = u(index_in) + du(index_in);

        cd_set_signal(SignalID, 0, u);
        exec;
        x = cd_get_signal(SignalID, 0, length(x));
        jac(:, index_in) = x;
        index_in = index_in + 1;
    end
    cd_set_signal(SignalID, 0, u0);
    exec;
    x = cd_get_signal(SignalID, 0, length(x));

    index_out = 1;
    while index_out <= Nout
        jac(index_out, :) = jac(index_out, :) - x(index_out);
        index_out = index_out + 1;
    end
    index_in = 1;
    while index_in <= Nin
        jac(:,index_in) = jac(:,index_in) / du(index_in);
        index_in = index_in + 1;
    end
    
    % find next u0
    u0 = u0 - inv(jac)*(x - xdes);
end

% find final value for x if needed
cd_set_signal(SignalID, 0, u0);
exec;
xfin = cd_get_signal(SignalID, 0, length(xfin));
ufin = u0;

== matlab function Vehicle Models/Quad-Rotor Model (Momentum)/Wash Coupling/Wash Coupling ==
  data: d input double; vw_omw output double; R input double; ROT_radius input double size=1; wind input double
function vw_omw  = wash_coupling(d, R, ROT_radius, wind)
% This block supports the Embedded MATLAB subset.
% See the help menu for details. 

ROT1  =  1:3;
ROT2  =  4:6;
ROT3  =  7:9;
ROT4  = 10:12;
FUSE  = 13:15;

ROT1v =  1:3;
ROT2v =  7:9;
ROT3v = 13:15;
ROT4v = 19:21;
FUSEv = 25:27;
vw_omw = zeros(30,1);

% Self-influence
vw_omw(ROT1v) = d(ROT1);
vw_omw(ROT2v) = d(ROT2);
vw_omw(ROT3v) = d(ROT3);
vw_omw(ROT4v) = d(ROT4);
vw_omw(FUSEv) = zeros(3,1);  % the fuselage model already has the self-influence included

% Main rotor on fuselage
% dist = sqrt((R(MR) - R(FUSE))' * (R(MR) - R(FUSE)));
% zor = dist / MR_radius;
% coef1 = 1 + zor / sqrt(1 + zor^2);
% vw_omw(FUSEv(3)) = vw_omw(FUSEv(3)) + coef1 * d(MR(3));

% Main rotor on horizontal stabilizer - assumes
% the horizontal stabilizer is always in the wake.
% dist = sqrt((R(MR) - R(HW))' * (R(MR) - R(HW)));
% zor = dist / MR_radius;
% coef1 = 1 + zor / sqrt(1 + zor^2);
% vw_omw(HWv(3)) = vw_omw(HWv(3)) + coef1 * d(MR(3));

% Fuselage on main rotor
% vw_omw(MRv(3)) = vw_omw(MRv(3)) + d(FUSE(3));

% Wind
vw_omw(ROT1v) = vw_omw(ROT1v) + wind;
vw_omw(ROT2v) = vw_omw(ROT2v) + wind;
vw_omw(ROT3v) = vw_omw(ROT3v) + wind;
vw_omw(ROT4v) = vw_omw(ROT4v) + wind;
vw_omw(FUSEv) = vw_omw(FUSEv) + wind;

% no rotation wakes generated

== matlab function Vehicle Models/Quad-Rotor Model (Momentum)/Fuselage/Fuselage Model (IERA)/Fuselage Forces and Moments/Fuselage Forces and Moments ==
  data: Parameters input Bus: FuselageParameters size=1; Environment input Bus: Environment size=1; FM_A output double size=6; va input double size=3; oma input double size=3
function FM_A  = fuselage_FM(Parameters, Environment, va, oma)
% Modeling of the fuselage forces and moments

% coef = [Parameters.cx'; Parameters.cy'; Parameters.cz'; 0 0 0; Parameters.cm'; Parameters.cn'];

% Calculate the aerodynamic forces and moments.
% fact1 = 0.5 * Environment.rho * Parameters.carea * va(1);
% fact2 = fact1 * Parameters.clen;
% FM_A = coef * va;
% FM_A(1:3) = FM_A(1:3) * fact1;
% FM_A(4:6) = FM_A(4:6) * fact2;

vfp = sqrt(va' * va);
if vfp > 0.0001
    alphaw = atan2(va(3), va(1));
    betaw = asin(va(2) / vfp);
    qtot = Environment.rho * vfp^2 / 2;
    Xf = -(20 + 30*sin(alphaw)^2) * qtot;
    Yf = (-200 * sin(betaw)) * qtot;
    Zf = -(-5 + 340*sin(alphaw)) * qtot;
    Lf = 0;
    Mf = (-100 + 2000*sin(alphaw)) * qtot;
    Nf = (-1000 * sin(betaw)) * qtot;
    FM_A = [Xf; Yf; Zf; Lf; Mf; Nf];
else
    FM_A = zeros(6,1);
end

FM_A = zeros(6,1);

== matlab function Vehicle Models/Quad-Rotor Model (Momentum)/Fuselage/Fuselage Model (IERA)/Fuselage Self-Influence/Fuselage Wash Self-Influence ==
  data: Parameters input Bus: FuselageParameters size=1; Environment input Bus: Environment size=1; d output double size=3; va input double size=3; oma input double size=3; FM_A input double size=6
function d  = fuselage_wash(Parameters, Environment, va, oma, FM_A)
% Fuselage Self-Influence
% Implements the equation 12.25

vatot = sqrt(va' * va);
if vatot < 0.0001
    d = [0; 0; 0];
else
    rtworho = -1 / (2 * Environment.rho * vatot);
    a11 = 0.002;
    a22 = 0.005;
    a33 = 0.003;
    d = rtworho * diag([a11 a22 a33]) * FM_A(1:3);
end

== matlab function Subsystem Models/Fin/Fin Model (IERA)/Fin/Fin Forces and Moments/Fin Forces and Moments (WRA axes) ==
  data: Parameters input Bus: FinParameters size=1; Environment input Bus: Environment size=1; FM_A output double size=6; va input double size=3; oma input double size=3
function FM_A  = fin_FM(Parameters, Environment, va, oma)
% Modeling of the fin forces and moments

%   Calculate some intermediate fin constants.
slambda = Parameters.taper;
b = Parameters.span;
croot = Parameters.chord;
s12 = b * croot * (1 + slambda) / 4;
stot = s12 * 2;
cbar = 2 * croot * (slambda^2 + slambda + 1) / 3 / (slambda + 1);
ar = b^2 / stot;
a03d_coef = ar / (ar + 2 * (ar + 4) / (ar + 2));

%   Calculate aerodynamic loads in WRA
aoa = atan2(va(3), va(1));

a = aoa - fix(aoa/pi)*pi;
if a > pi/2
    a = -pi+a;
end
if a < -pi/2
    a = pi+a;
end

if abs(a) > Parameters.stall + 5*pi/180
    cl = Parameters.a1s2 * sin(2*a);
elseif abs(a) >=Parameters. stall
    k = (abs(a) - Parameters.stall) / (5*pi/180);
    cl = (1-k) * Parameters.a0 * a  + k * Parameters.a1s2 * sin(2*a);
else
    cl = Parameters.a0 * a;
end
cl = a03d_coef * cl;

cd = Parameters.cd0 + Parameters.cd1s1 * sin(aoa) + Parameters.cd2c1 * cos(aoa)^2;
cm = Parameters.cm0 + Parameters.cm1s1 * sin(aoa);

v2 = va'*va;
qtots = Environment.rho * v2 / 2 * stot;
drag = qtots * cd;
lift = qtots * cl;
momy = qtots * cbar * cm;
F = [-drag; 0; -lift];
M = [0; momy; 0];
Tt = [ cos(-aoa) 0 -sin(-aoa); 0 1 0; sin(-aoa) 0 cos(-aoa)];
FM_A = [Tt' * F; Tt' * M];

== matlab function Subsystem Models/Fin/Fin Model (IERA)/Fin Self-Influence/Fin Wash Self-Influence (IERA) ==
  data: Parameters input Bus: FinParameters size=1; Environment input Bus: Environment size=1; d output double size=3; va input double size=3; oma input double size=3; FM_A input double size=6
function d  = fin_wash(Parameters, Environment, va, oma, FM_A)
% Wing Self-Influence
% Implements the equation 12.12

vatot = sqrt(va' * va);
if vatot < 0.0001
    d = [0; 0; 0];
else
    rtworho = -1 / (2 * Environment.rho * vatot);
    a11 = 4 / (pi * Parameters.span^2);
    a22 = a11;
    a33 = a11;
    d = rtworho * diag([a11 a22 a33]) * FM_A(1:3);
end

== matlab function Subsystem Models/Fuselage/Fuselage Model (IERA)/Fuselage Forces and Moments/Fuselage Forces and Moments ==
  data: Parameters input Bus: FuselageParameters size=1; Environment input Bus: Environment size=1; FM_A output double size=6; va input double size=3; oma input double size=3
function FM_A  = fuselage_FM(Parameters, Environment, va, oma)
% Modeling of the fuselage forces and moments

% coef = [Parameters.cx'; Parameters.cy'; Parameters.cz'; 0 0 0; Parameters.cm'; Parameters.cn'];

% Calculate the aerodynamic forces and moments.
% fact1 = 0.5 * Environment.rho * Parameters.carea * va(1);
% fact2 = fact1 * Parameters.clen;
% FM_A = coef * va;
% FM_A(1:3) = FM_A(1:3) * fact1;
% FM_A(4:6) = FM_A(4:6) * fact2;

vfp = sqrt(va' * va);
if vfp > 0.0001
    alphaw = atan2(va(3), va(1));
    betaw = asin(va(2) / vfp);
    qtot = Environment.rho * vfp^2 / 2;
    Xf = -(20 + 30*sin(alphaw)^2) * qtot;
    Yf = (-200 * sin(betaw)) * qtot;
    Zf = -(-5 + 340*sin(alphaw)) * qtot;
    Lf = 0;
    Mf = (-100 + 2000*sin(alphaw)) * qtot;
    Nf = (-1000 * sin(betaw)) * qtot;
    FM_A = [Xf; Yf; Zf; Lf; Mf; Nf];
else
    FM_A = zeros(6,1);
end

== matlab function Subsystem Models/Fuselage/Fuselage Model (IERA)/Fuselage Self-Influence/Fuselage Wash Self-Influence ==
  data: Parameters input Bus: FuselageParameters size=1; Environment input Bus: Environment size=1; d output double size=3; va input double size=3; oma input double size=3; FM_A input double size=6
function d  = fuselage_wash(Parameters, Environment, va, oma, FM_A)
% Fuselage Self-Influence
% Implements the equation 12.25

vatot = sqrt(va' * va);
if vatot < 0.0001
    d = [0; 0; 0];
else
    rtworho = -1 / (2 * Environment.rho * vatot);
    a11 = 0.002;
    a22 = 0.005;
    a33 = 0.003;
    d = rtworho * diag([a11 a22 a33]) * FM_A(1:3);
end

== matlab function Subsystem Models/Helicopter Rotor/Rotor Model (IERA)/Rotor Flapping/Rotor Flapping (Wind-Mast axes) ==
  data: Parameters input Bus: RotorParameters size=1; Environment input Bus: Environment size=1; vi input double size=3; omi input double size=3; vid input double size=3; omid input double size=3; flap_dot output double size=3; va input double size=3; oma input double size=3; flap input double size=3; cz input double size=1; controls input double size=3; omega input double size=1; flap_static output double size=3
function [flap_dot,flap_static] = rotor_flapping(Parameters, Environment, vi, omi, vid, omid, va, oma, flap, cz, controls, omega)
% Dynamic modeling of the rotor flapping
% Implements equations 11.52, K.7
%   controls (3x1) = [theta0 A1 B1]' are the rotor control inputs
%   omega is the rotor rotation speed in body axes
%   va (3x1), oma (3x1), flap, bt, eps0 are initial conditions

if Parameters.iflap
    iflap = Parameters.iflap;
else
    iflap = Parameters.mbar * Parameters.radius^3 / 3;
end
if Parameters.mbar
    m1 = Parameters.mbar * Parameters.radius^2 / 2;
else
    m1 = Parameters.iflap / Parameters.radius * 3/2;
end
gamma = Environment.rho * Parameters.chord * Parameters.a0 * Parameters.radius^4 / iflap;
sigma = double(Parameters.nb) * Parameters.chord / (pi * Parameters.radius);
prev = sqrt(1 + 3 * Parameters.e / (2 * (Parameters.radius - Parameters.e)) + ...
       Parameters.khub / (iflap * omega^2) + gamma * tan(Parameters.delta3) / 8);
bt = 1 - sqrt(2 * abs(cz)) / double(Parameters.nb);
bt = max([min([bt Parameters.btmax]) Parameters.btmin]);
clbar = -6 * cz / sigma;
cdavg = Parameters.del0_2(1) + clbar * (Parameters.del0_2(2) + clbar * Parameters.del0_2(3));
eps0 = cdavg / Parameters.a0;

bt2 = bt  * bt;
bt3 = bt2 * bt;
bt4 = bt3 * bt;
bt5 = bt4 * bt;
omegap = omega - omi(3);
omegaa = omega - oma(3);
vtipa = omegaa * Parameters.radius;
mu = va(1) / vtipa;
lambda = va(3) / vtipa;
pahat = oma(1) / omegaa;
qahat = oma(2) / omegaa;
pihat = omi(1) / omegap;
qihat = omi(2) / omegap;
pid = omid(1);
qid = omid(2);
ax = vid(1);
ay = vid(2);
az = vid(3);

% controls
theta0 = controls(1);
A1 = controls(2);
B1 = controls(3);
%flapping
beta0 = (flap(1) - Parameters.precone) * double(Parameters.hubtype) + Parameters.precone;
a1 = flap(2);
b1 = flap(3);

fom = omegaa / omegap;
fom2 = fom^2;

db0b0d = (bt4 / 4) * fom;
db0b1d = (bt3 * mu / 6) * fom;
da1b0d = (bt3 * mu / 3) * fom;
da1b1d = (bt4 / 4) * fom;
db1a1d = (bt4 / 4) * fom;

f0 = (bt4 / 4 + bt2 * mu^2 / 4) * fom2;
ft = (bt5 / 5 + bt3 * mu^2 / 6) * fom2;
fla = (bt3 / 3) * (1 + eps0) * fom2;
fcb1 = (bt3 * mu / 3) * fom2;
fp = (bt3 * mu / 6) * (1 + eps0) * fom2;
fa1 = (bt3 * mu / 6 / fom) * (1 + eps0) * (1 - fom) * fom2;

aa0 = (2 * bt3 * mu / 3) * fom2;
aat = (bt4 * mu / 2) * fom2;
aala = (bt2 * mu / 2 - mu^3 / 8) * (1 + eps0) * fom2;
aacb1 = (bt4 / 4 + 3 * bt2 * mu^2 / 8) * fom2;
aap = (bt4 / 4) * (1 + eps0) * fom2;
aa1 = (bt4 / 4 / fom - bt2 * mu^2 / 8) * (1 + eps0) * fom2;

bb0 = (bt3 * mu / 3) * (1 + eps0) * fom2;
bca1 = (bt4 / 4 + bt2 * mu^2 / 8) * fom2;
bq = (bt4 / 4) * (1 + eps0) * fom2;
bb1 = (bt4 / 4 / fom + bt2 * mu^2 / 8) * (1 + eps0) * fom2;

fdmtx = zeros(3, 3);
fdmtx(1, 1) = gamma * db0b0d / 2 / omegap;
fdmtx(1, 2) = 0;
fdmtx(1, 3) = -gamma * db0b1d / 2 / omegap;
fdmtx(2, 1) = gamma * da1b0d / 2 / omegap;
fdmtx(2, 2) = 2 / omegap;
fdmtx(2, 3) = -gamma * da1b1d / 2 / omegap;
fdmtx(3, 1) = 0;
fdmtx(3, 2) = -gamma * db1a1d / 2 / omegap;
fdmtx(3, 3) = -2 / omegap;

fmtx = zeros(3, 3);
fmtx(1, 1) = prev^2;
fmtx(1, 2) = gamma * fa1 / 2;
fmtx(1, 3) = 0;
fmtx(2, 1) = 0;
fmtx(2, 2) = gamma * aa1 / 2;
fmtx(2, 3) = 1 - prev^2;
fmtx(3, 1) = gamma * bb0 / 2;
fmtx(3, 2) = 1 - prev^2;
fmtx(3, 3) = -gamma * bb1 / 2;

cmtx = zeros(3, 4);
cmtx(1, 1) = gamma * f0 / 2;
cmtx(1, 2) = gamma * ft / 2;
cmtx(1, 3) = 0;
cmtx(1, 4) = gamma * fcb1 / 2;
cmtx(2, 1) = gamma * aa0 / 2;
cmtx(2, 2) = gamma * aat / 2;
cmtx(2, 3) = 0;
cmtx(2, 4) = gamma * aacb1 / 2;
cmtx(3, 1) = 0;
cmtx(3, 2) = 0;
cmtx(3, 3) = gamma * bca1 / 2;
cmtx(3, 4) = 0;

rmtx = zeros(3, 3);
rmtx(1, 1) = gamma * fla / 2;
rmtx(1, 2) = gamma * fp / 2;
rmtx(1, 3) = 0;
rmtx(2, 1) = gamma * aala / 2;
rmtx(2, 2) = gamma * aap / 2;
rmtx(2, 3) = 0;
rmtx(3, 1) = 0;
rmtx(3, 2) = 0;
rmtx(3, 3) = gamma * bq / 2;

acmtx = zeros(3, 7);
acmtx(1, 1) = 0;
acmtx(1, 2) = 0;
acmtx(1, 3) = 0;
acmtx(1, 4) = 0;
acmtx(1, 5) = -m1 * Parameters.radius * a1 / 2 / iflap;
acmtx(1, 6) = m1 * Parameters.radius * b1 / 2 / iflap;
acmtx(1, 7) = m1 * Parameters.radius / iflap;
acmtx(2, 1) = 0;
acmtx(2, 2) = -2;
acmtx(2, 3) = 1;
acmtx(2, 4) = 0;
acmtx(2, 5) = 0;
acmtx(2, 6) = -m1 * Parameters.radius * beta0 / iflap;
acmtx(2, 7) = 0;
acmtx(3, 1) = 2;
acmtx(3, 2) = 0;
acmtx(3, 3) = 0;
acmtx(3, 4) = 1;
acmtx(3, 5) = m1 * Parameters.radius * beta0 / iflap;
acmtx(3, 6) = 0;
acmtx(3, 7) = 0;

cvec  = [theta0; Parameters.twist; A1; B1];
rvec  = [lambda; pahat; qahat];
acvec = [pihat; qihat; [pid; qid]/(omegap^2); [ax; ay; az]/(Parameters.radius*omegap^2)];

% calculate RHS of 11.52
RHS = acmtx * acvec + rmtx * rvec + cmtx * cvec;
% static flapping for trimming
flap_static = inv(fmtx) * RHS;
flap_static(1) = (flap_static(1) - Parameters.precone) * double(Parameters.hubtype) + Parameters.precone;
% first order dynamic flapping
flap_dot = inv(fdmtx) * (RHS - fmtx * flap);
